simulink model "Control_PID_con_Perturbaciones"  (R2025b)
settings: Solver=ode45  StartTime=0.0  StopTime=30  RelTol=1e-3
libraries: slpidlib x1
settings Model: Creator=Carlo  LastModifiedBy=Carlo
settings DataIOCC: SaveState=on

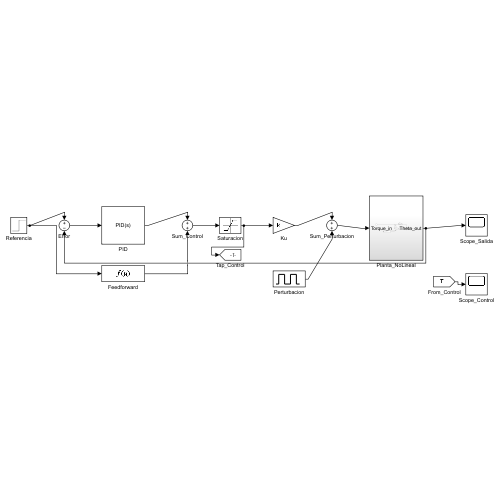
[thumbnail: Simulink's stored preview of the top-level diagram]
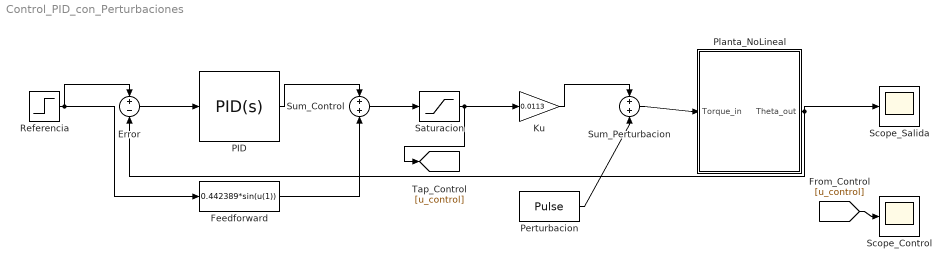
== system Control_PID_con_Perturbaciones ==
  Error : Sum  Inputs=+-
  Feedforward : Fcn  Expr=0.442389*sin(u(1))
  Ku : Gain  Gain=0.0113
  PID : slpidlib/PID Controller  Controller=PID  Form=Parallel  TimeDomain=Continuous-time  UseExternalTs=off  SampleTime=-1  IntegratorMethod=Forward Euler  FilterMethod=Forward Euler  ControllerParametersSource=internal  P=0.98857  I=4.0707  UseKiTs=off  D=3.5088  UseExternalDerivativeSource=off  N=20  UseFilter=on  TunerSelectOption=Transfer Function Based (PID Tuner App)  InitialConditionSource=internal  InitialConditionForIntegrator=0  InitialConditionForFilter=0  DifferentiatorICPrevScaledInput=0  ExternalReset=none  TrackingMode=off  Kt=1  LimitOutput=off  SatLimitsSource=internal  UpperSaturationLimit=inf  LowerSaturationLimit=-inf  LinearizeAsGain=on  AntiWindupMode=none  Kb=2.8571  LimitIntegrator=off  UpperIntegratorSaturationLimit=inf  LowerIntegratorSaturationLimit=-inf  POutMin=[]  POutMax=[]  IOutMin=[]  IOutMax=[]  DOutMin=[]  DOutMax=[]  NOutMin=[]  NOutMax=[]  SumOutMin=[]  SumOutMax=[]  SaturationOutMin=[]  SaturationOutMax=[]  PParamMin=[]  PParamMax=[]  IParamMin=[]  IParamMax=[]  DParamMin=[]  DParamMax=[]  NParamMin=[]  NParamMax=[]  KbParamMin=[]  KbParamMax=[]  KtParamMin=[]  KtParamMax=[]  KbOutMin=[]  KbOutMax=[]  KtOutMin=[]  KtOutMax=[]  IntegratorOutMin=[]  IntegratorOutMax=[]  FilterOutMin=[]  FilterOutMax=[]  SumI1OutMin=[]  SumI1OutMax=[]  SumI2OutMin=[]  SumI2OutMax=[]  SumI3OutMin=[]  SumI3OutMax=[]  SumI4OutMin=[]  SumI4OutMax=[]  SumDOutMin=[]  SumDOutMax=[]  DifferentiatorOutMin=[]  DifferentiatorOutMax=[]  FilterDiffOutCoefMin=[]  FilterDiffOutCoefMax=[]  ReciprocalOutMin=[]  ReciprocalOutMax=[]  SumDenOutMin=[]  SumDenOutMax=[]  SumNumOutMin=[]  SumNumOutMax=[]  DivideOutMin=[]  DivideOutMax=[]  UdiffTsProdOutMin=[]  UdiffTsProdOutMax=[]  NTsProdOutMin=[]  NTsProdOutMax=[]  UintegralTsProdOutMin=[]  UintegralTsProdOutMax=[]  UngainTsProdOutMin=[]  UngainTsProdOutMax=[]  ClampingZeroOutDataTypeStr=Inherit: Inherit via back propagation  ClampingZeroOutMin=[]  ClampingZeroOutMax=[]  FilterDenConstantOutDataTypeStr=Inherit: Inherit via back propagation  FilterDenConstantOutMin=[]  FilterDenConstantOutMax=[]  PCopyOutDataTypeStr=Inherit: Inherit via back propagation  PCopyOutMin=[]  PCopyOutMax=[]  NCopyOutDataTypeStr=Inherit: Inherit via back propagation  NCopyOutMin=[]  NCopyOutMax=[]  IntegratorContinuousStateAttributes=''  IntegratorStateMustResolveToSignalObject=off  IntegratorRTWStateStorageClass=Auto  FilterContinuousStateAttributes=''  FilterStateMustResolveToSignalObject=off  FilterRTWStateStorageClass=Auto  ParallelPVariant=InternalParameters  IdealPVariant=Disabled  IVariant=InternalParameters  DVariant=InternalParameters  IntegratorVariant=Continuous  SatVariant=Disabled  AWVariant=Passthrough  PCopyVariant=Disabled  TRVariant=Disabled  FdbkBlocksVariant=Forward  IdealPFdbkVariant=Disabled  SatFdbkVariant=Disabled  DerivativeFilterVariant=ContFilter  NVariant=InternalParameters  NCopyVariant=Disabled  FilterICVariant=InternalICsFilter  IntegratorICVariant=InternalICs  ExternalResetVariant=Disabled  TRSumVariant=Passthrough  SumFdbkVariant=Disabled  SumVariant=Sum_PID  TsampFilterVariant=InternalTs  TsampNgainVariant=Passthrough  TsampIntegralVariant=Disabled_SignalSpec  ExternalSaturationOutDataTypeStr=Inherit: Same as second input  DerivativeSourceVariant=ErrorSignal  PreIntVariant=InternalPreInt
  Perturbacion : DiscretePulseGenerator  PulseType=Time based  Amplitude=0.002  Period=3  PulseWidth=20
  Planta_NoLineal : Subsystem
  Referencia : Step  Time=0  After=0.87266  SampleTime=0
  Saturacion : Saturate  UpperLimit=1  LowerLimit=-1
  Scope_Control : Scope
      settings: ActiveDisplayYMinimum=0.0935756496598949  ActiveDisplayYMaximum=0.41456363428830739
  Scope_Salida : Scope
      settings: ActiveDisplayYMinimum=0.85046003073746668  ActiveDisplayYMaximum=0.90242872962076159
  Sum_Control : Sum
  Sum_Perturbacion : Sum
  wires:
  Referencia/1 -> Error/1, Feedforward/1
  Error/1 -> PID/1
  PID/1 -> Sum_Control/1
  Sum_Control/1 -> Saturacion/1
  Saturacion/1 -> Ku/1, [u_control]
  Ku/1 -> Sum_Perturbacion/1
  Perturbacion/1 -> Sum_Perturbacion/2
  Sum_Perturbacion/1 -> Planta_NoLineal/1(Torque_in)
  Planta_NoLineal/1(Theta_out) -> Scope_Salida/1, Error/2
  Feedforward/1 -> Sum_Control/2
  [u_control] -> Scope_Control/1

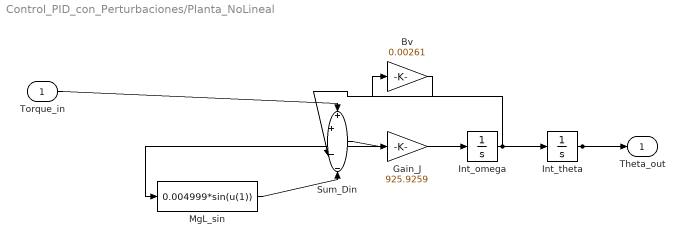
== system Control_PID_con_Perturbaciones/Planta_NoLineal ==
  Torque_in : Inport
  Bv : Gain  Gain=0.00261
  Gain_J : Gain  Gain=925.9259
  Int_omega : Integrator
  Int_theta : Integrator  InitialCondition=0.87266
  MgL_sin : Fcn  Expr=0.004999*sin(u(1))
  Sum_Din : Sum  Inputs=++--
  Theta_out : Outport
  wires:
  Torque_in/1 -> Sum_Din/1
  Sum_Din/1 -> Gain_J/1
  Gain_J/1 -> Int_omega/1
  Int_omega/1 -> Int_theta/1, Bv/1
  Int_theta/1 -> Theta_out/1, MgL_sin/1
  MgL_sin/1 -> Sum_Din/4
  Bv/1 -> Sum_Din/3
